simulink model "brayton_cycle_lstm_simplified_compare"  (R2023a)
settings: Solver=ode23t  StartTime=0.0  StopTime=100  RelTol=1e-3
PreLoadFcn:
  | combustor_volume = 0.001; % m^3
  | flow_area = 0.002; % m^2;
  | shaft_inertia = 0.1; % kg*m^2
  | mechanical_efficiency = 0.98; % 1
  | apu_shaft_speed = 6000; % rpm
  | 
  | % Compressor Map
  | 
  | compressor.beta_vector = [
  |      0, 0.1, 0.2, 0.3, 0.4, 0.5, 0.6, 0.7, 0.8, 0.9, 1.0];
  | 
  | compressor.corrected_speed_vector = [
  |     5000, 6000, 7000, 8000, 8500, 9000, 9500, 10000, 11000, 12000
  |     ]; % rpm
  | 
  | compressor.map.pressure_ratio = [
  |     0.1806    0.4817    0.8258    1.1561    1.4451    1.7002    2.0645    2.4086    2.6275    2.7527    2.8903
  |     0.2364    0.6303    1.0806    1.5128    1.8910    2.2247    2.7014    3.1517    3.4382    3.6019    3.7820
  |     0.2921    0.7790    1.3354    1.8695    2.3369    2.7493    3.3384    3.8948    4.2489    4.4512    4.6738
  |     0.4031    1.0748    1.8425    2.5795    3.2244    3.7934    4.6063    5.3740    5.8625    6.1417    6.4488
  |     0.5503    1.4673    2.5155    3.5216    4.4021    5.1789    6.2886    7.3368    8.0037    8.3849    8.8041
  |     0.7404    1.9745    3.3849    4.7388    5.9235    6.9688    8.4621    9.8725   10.7700   11.2829   11.8470
  |     0.9903    2.6407    4.5270    6.3378    7.9222    9.3203   11.3175   13.2037   14.4041   15.0900   15.8445
  |     1.2261    3.2697    5.6051    7.8472    9.8090   11.5400   14.0129   16.3483   17.8345   18.6838   19.6180
  |     1.2827    3.4206    5.8639    8.2094   10.2617   12.0726   14.6596   17.1029   18.6577   19.5462   20.5235
  |     1.3393    3.5715    6.1226    8.5716   10.7145   12.6053   15.3064   17.8575   19.4809   20.4086   21.4290]; % 1
  | 
  | compressor.map.corrected_mass_flow_rate = [
  |     0.0400    0.0400    0.0400    0.0399    0.0395    0.0389    0.0378    0.0363    0.0349    0.0340    0.0329
  |     0.0530    0.0530    0.0530    0.0527    0.0521    0.0513    0.0501    0.0481    0.0462    0.0449    0.0434
  |     0.0640    0.0640    0.0639    0.0635    0.0630    0.0623    0.0611    0.0589    0.0565    0.0549    0.0530
  |     0.1000    0.1000    0.0997    0.0991    0.0983    0.0974    0.0951    0.0906    0.0870    0.0846    0.0814
  |     0.1350    0.1350    0.1346    0.1340    0.1332    0.1324    0.1301    0.1258    0.1222    0.1197    0.1165
  |     0.1700    0.1699    0.1695    0.1688    0.1681    0.1673    0.1654    0.1620    0.1589    0.1562    0.1521
  |     0.2100    0.2097    0.2089    0.2077    0.2064    0.2051    0.2021    0.1978    0.1925    0.1882    0.1824
  |     0.2500    0.2498    0.2494    0.2488    0.2480    0.2472    0.2452    0.2414    0.2375    0.2338    0.2287
  |     0.2600    0.2599    0.2595    0.2589    0.2581    0.2574    0.2555    0.2516    0.2482    0.2453    0.2415
  |     0.2640    0.2639    0.2635    0.2629    0.2622    0.2616    0.2604    0.2580    0.2558    0.2542    0.2513]; % kg/s
  | 
  | compressor.map.efficiency = [
  |     0.3500    0.4200    0.4900    0.5600    0.5950    0.6300    0.6650    0.6860    0.6650    0.5600    0.4900
  |     0.3600    0.4320    0.5040    0.5760    0.6120    0.6480    0.6840    0.7056    0.6840    0.5760    0.5040
  |     0.3750    0.4500    0.5250    0.6000    0.6375    0.6750    0.7125    0.7350    0.7125    0.6000    0.5250
  |     0.3900    0.4680    0.5460    0.6240    0.6630    0.7020    0.7410    0.7644    0.7410    0.6240    0.5460
  |     0.4000    0.4800    0.5600    0.6400    0.6800    0.7200    0.7600    0.7840    0.7600    0.6400    0.5600
  |     0.4250    0.5100    0.5950    0.6800    0.7225    0.7650    0.8075    0.8330    0.8075    0.6800    0.5950
  |     0.4500    0.5400    0.6300    0.7200    0.7650    0.8100    0.8550    0.8820    0.8550    0.7200    0.6300
  |     0.4900    0.5880    0.6860    0.7840    0.8330    0.8820    0.9310    0.9604    0.9310    0.7840    0.6860
  |     0.4500    0.5400    0.6300    0.7200    0.7650    0.8100    0.8550    0.8820    0.8550    0.7200    0.6300
  |     0.4000    0.4800    0.5600    0.6400    0.6800    0.7200    0.7600    0.7840    0.7600    0.6400    0.5600]; % 1
  | 
  | compressor.reference_pressure = 0.101325; % MPa
  | compressor.reference_temperature = 288.15; % K
  | 
  | % Turbine Map
  | 
  | turbine.flow_map.pressure_ratio = [
  |     1.0010, 1.0050, 1.0101, 1.0204, 1.0309, 1.0417, 1.0526, 1.1111, 1.1765, 1.2500, 1.3333, 1.4286, 1.5385, 1.6667, 1.8182, 2.0000
  |     ]; %  1
  | turbine.flow_map.corrected_mass_flow_rate = [
  | ... (+17 lines)
model workspace (MAT data in the model file):
  rpm0 = 4800
  rpm_setpoint = [4000 4000 5000 5000 6000 6000 7000 7000 8000 8000 9000 9000 ... (19 elements, 1x19)]
  time_setpoint = [0 200 220 300 320 400 420 500 520 600 620 700 ... (19 elements, 1x19)]
undefined symbols (not defined in the file or in its folder): ix, scenario
libraries: fl_lib x32, nesl_utility x10, simulink x4, SimscapeFluids_lib x3, slpidlib x3, deeplib x3, SignalEditorBlockLib x1
(part 2 of 2)

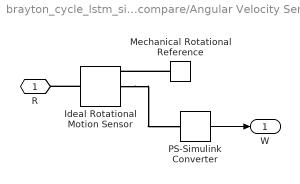
== system brayton_cycle_lstm_simplified_compare/Angular Velocity Sensor ==
  Ideal Rotational Motion Sensor : fl_lib/Mechanical/Mechanical Sensors/Ideal Rotational Motion Sensor  reference=foundation.enum.MeasurementReference.difference  acceleration_port=false  velocity_port=true  position_port=true  wrap_angle=simscape.enum.onoff.off  offset=0 rad
  Mechanical Rotational Reference : fl_lib/Mechanical/Rotational Elements/Mechanical Rotational Reference
  PS-Simulink Converter : nesl_utility/PS-Simulink Converter  PhysicalDomain=network_engine_domain  SubClassName=ps_output  LeftPortType=input  RightPortType=output  PseudoPeriodic=off  Frequencies=[]  VectorFormat=1-D array  Unit=rpm  AffineConversion=off
  R : PMIOPort  Side=Left
  W : Outport  VectorParamsAs1DForOutWhenUnconnected=off
  wires:
  PS-Simulink Converter/1 -> W/1
  connections:
  Ideal Rotational Motion Sensor/LConn1 -- R/RConn1
  Ideal Rotational Motion Sensor/RConn2 -- PS-Simulink Converter/LConn1
  Mechanical Rotational Reference/LConn1 -- Ideal Rotational Motion Sensor/RConn1

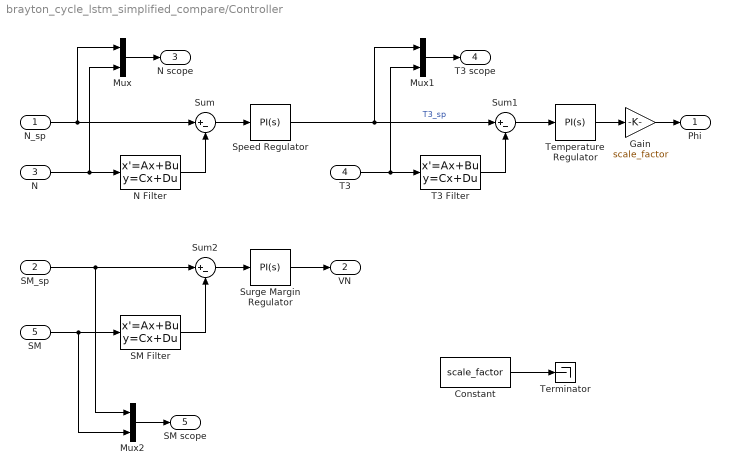
== system brayton_cycle_lstm_simplified_compare/Controller ==
  N_sp : Inport
  SM_sp : Inport  Port=2
  N : Inport  Port=3
  T3 : Inport  Port=4
  SM : Inport  Port=5
  Constant : Constant  Value=scale_factor
  Gain : Gain  Gain=scale_factor
  Mux : Mux  Inputs=2
  Mux1 : Mux  Inputs=2
  Mux2 : Mux  Inputs=2
  N Filter : StateSpace  A=-100  B=100  D=0  InitialCondition=10000
  SM Filter : StateSpace  A=-100  B=100  D=0  InitialCondition=0.25
  Speed Regulator : slpidlib/PID Controller  Controller=PI  Form=Ideal  TimeDomain=Continuous-time  UseExternalTs=off  SampleTime=-1  IntegratorMethod=Forward Euler  FilterMethod=Forward Euler  ControllerParametersSource=internal  P=0.5  I=1  UseKiTs=off  D=0  N=100  UseFilter=on  TunerSelectOption=Transfer Function Based (PID Tuner App)  InitialConditionSource=internal  InitialConditionForIntegrator=273.15  InitialConditionForFilter=0  DifferentiatorICPrevScaledInput=0  ExternalReset=none  TrackingMode=off  Kt=1  LimitOutput=on  SatLimitsSource=internal  UpperSaturationLimit=1800  LowerSaturationLimit=273.15  LinearizeAsGain=on  AntiWindupMode=back-calculation  Kb=1/0.5  LimitIntegrator=off  UpperIntegratorSaturationLimit=inf  LowerIntegratorSaturationLimit=-inf  POutMin=[]  POutMax=[]  IOutMin=[]  IOutMax=[]  DOutMin=[]  DOutMax=[]  NOutMin=[]  NOutMax=[]  SumOutMin=[]  SumOutMax=[]  SaturationOutMin=[]  SaturationOutMax=[]  PParamMin=[]  PParamMax=[]  IParamMin=[]  IParamMax=[]  DParamMin=[]  DParamMax=[]  NParamMin=[]  NParamMax=[]  KbParamMin=[]  KbParamMax=[]  KtParamMin=[]  KtParamMax=[]  KbOutMin=[]  KbOutMax=[]  KtOutMin=[]  KtOutMax=[]  IntegratorOutMin=[]  IntegratorOutMax=[]  FilterOutMin=[]  FilterOutMax=[]  SumI1OutMin=[]  SumI1OutMax=[]  SumI2OutMin=[]  SumI2OutMax=[]  SumI3OutMin=[]  SumI3OutMax=[]  SumI4OutMin=[]  SumI4OutMax=[]  SumDOutMin=[]  SumDOutMax=[]  DifferentiatorOutMin=[]  DifferentiatorOutMax=[]  FilterDiffOutCoefMin=[]  FilterDiffOutCoefMax=[]  ReciprocalOutMin=[]  ReciprocalOutMax=[]  SumDenOutMin=[]  SumDenOutMax=[]  SumNumOutMin=[]  SumNumOutMax=[]  DivideOutMin=[]  DivideOutMax=[]  UdiffTsProdOutMin=[]  UdiffTsProdOutMax=[]  NTsProdOutMin=[]  NTsProdOutMax=[]  UintegralTsProdOutMin=[]  UintegralTsProdOutMax=[]  UngainTsProdOutMin=[]  UngainTsProdOutMax=[]  ClampingZeroOutDataTypeStr=Inherit: Inherit via back propagation  ClampingZeroOutMin=[]  ClampingZeroOutMax=[]  FilterDenConstantOutDataTypeStr=Inherit: Inherit via back propagation  FilterDenConstantOutMin=[]  FilterDenConstantOutMax=[]  PCopyOutDataTypeStr=Inherit: Inherit via back propagation  PCopyOutMin=[]  PCopyOutMax=[]  NCopyOutDataTypeStr=Inherit: Inherit via back propagation  NCopyOutMin=[]  NCopyOutMax=[]  IntegratorContinuousStateAttributes=''  IntegratorStateMustResolveToSignalObject=off  IntegratorRTWStateStorageClass=Auto  FilterContinuousStateAttributes=''  FilterStateMustResolveToSignalObject=off  FilterRTWStateStorageClass=Auto  ParallelPVariant=Passthrough  IdealPVariant=InternalParameters  IVariant=InternalParameters  DVariant=Disabled  IntegratorVariant=Continuous  SatVariant=Enabled  AWVariant=BackCalculation  PCopyVariant=Disabled  TRVariant=Disabled  FdbkBlocksVariant=Forward  IdealPFdbkVariant=Disabled  SatFdbkVariant=Disabled  DerivativeFilterVariant=Disabled  NVariant=Disabled  NCopyVariant=Disabled_SignalSpec  FilterICVariant=Disabled  IntegratorICVariant=InternalICs  ExternalResetVariant=Disabled  TRSumVariant=Passthrough  SumFdbkVariant=Disabled  SumVariant=Sum_PI  TsampFilterVariant=InternalTs  TsampNgainVariant=Passthrough  TsampIntegralVariant=Disabled_SignalSpec  ExternalSaturationOutDataTypeStr=Inherit: Same as second input
  Sum : Sum  Inputs=|+-
  Sum1 : Sum  Inputs=|+-
  Sum2 : Sum  Inputs=|+-
  Surge Margin Regulator : slpidlib/PID Controller  Controller=PI  Form=Ideal  TimeDomain=Continuous-time  UseExternalTs=off  SampleTime=-1  IntegratorMethod=Forward Euler  FilterMethod=Forward Euler  ControllerParametersSource=internal  P=1  I=1  UseKiTs=off  D=0  N=100  UseFilter=on  TunerSelectOption=Transfer Function Based (PID Tuner App)  InitialConditionSource=internal  InitialConditionForIntegrator=0.15  InitialConditionForFilter=0  DifferentiatorICPrevScaledInput=0  ExternalReset=none  TrackingMode=off  Kt=1  LimitOutput=on  SatLimitsSource=internal  UpperSaturationLimit=1  LowerSaturationLimit=0.15  LinearizeAsGain=on  AntiWindupMode=back-calculation  Kb=1  LimitIntegrator=off  UpperIntegratorSaturationLimit=inf  LowerIntegratorSaturationLimit=-inf  POutMin=[]  POutMax=[]  IOutMin=[]  IOutMax=[]  DOutMin=[]  DOutMax=[]  NOutMin=[]  NOutMax=[]  SumOutMin=[]  SumOutMax=[]  SaturationOutMin=[]  SaturationOutMax=[]  PParamMin=[]  PParamMax=[]  IParamMin=[]  IParamMax=[]  DParamMin=[]  DParamMax=[]  NParamMin=[]  NParamMax=[]  KbParamMin=[]  KbParamMax=[]  KtParamMin=[]  KtParamMax=[]  KbOutMin=[]  KbOutMax=[]  KtOutMin=[]  KtOutMax=[]  IntegratorOutMin=[]  IntegratorOutMax=[]  FilterOutMin=[]  FilterOutMax=[]  SumI1OutMin=[]  SumI1OutMax=[]  SumI2OutMin=[]  SumI2OutMax=[]  SumI3OutMin=[]  SumI3OutMax=[]  SumI4OutMin=[]  SumI4OutMax=[]  SumDOutMin=[]  SumDOutMax=[]  DifferentiatorOutMin=[]  DifferentiatorOutMax=[]  FilterDiffOutCoefMin=[]  FilterDiffOutCoefMax=[]  ReciprocalOutMin=[]  ReciprocalOutMax=[]  SumDenOutMin=[]  SumDenOutMax=[]  SumNumOutMin=[]  SumNumOutMax=[]  DivideOutMin=[]  DivideOutMax=[]  UdiffTsProdOutMin=[]  UdiffTsProdOutMax=[]  NTsProdOutMin=[]  NTsProdOutMax=[]  UintegralTsProdOutMin=[]  UintegralTsProdOutMax=[]  UngainTsProdOutMin=[]  UngainTsProdOutMax=[]  ClampingZeroOutDataTypeStr=Inherit: Inherit via back propagation  ClampingZeroOutMin=[]  ClampingZeroOutMax=[]  FilterDenConstantOutDataTypeStr=Inherit: Inherit via back propagation  FilterDenConstantOutMin=[]  FilterDenConstantOutMax=[]  PCopyOutDataTypeStr=Inherit: Inherit via back propagation  PCopyOutMin=[]  PCopyOutMax=[]  NCopyOutDataTypeStr=Inherit: Inherit via back propagation  NCopyOutMin=[]  NCopyOutMax=[]  IntegratorContinuousStateAttributes=''  IntegratorStateMustResolveToSignalObject=off  IntegratorRTWStateStorageClass=Auto  FilterContinuousStateAttributes=''  FilterStateMustResolveToSignalObject=off  FilterRTWStateStorageClass=Auto  ParallelPVariant=Passthrough  IdealPVariant=InternalParameters  IVariant=InternalParameters  DVariant=Disabled  IntegratorVariant=Continuous  SatVariant=Enabled  AWVariant=BackCalculation  PCopyVariant=Disabled  TRVariant=Disabled  FdbkBlocksVariant=Forward  IdealPFdbkVariant=Disabled  SatFdbkVariant=Disabled  DerivativeFilterVariant=Disabled  NVariant=Disabled  NCopyVariant=Disabled_SignalSpec  FilterICVariant=Disabled  IntegratorICVariant=InternalICs  ExternalResetVariant=Disabled  TRSumVariant=Passthrough  SumFdbkVariant=Disabled  SumVariant=Sum_PI  TsampFilterVariant=InternalTs  TsampNgainVariant=Passthrough  TsampIntegralVariant=Disabled_SignalSpec  ExternalSaturationOutDataTypeStr=Inherit: Same as second input
  T3 Filter : StateSpace  A=-100  B=100  D=0  InitialCondition=288.15
  Temperature Regulator : slpidlib/PID Controller  Controller=PI  Form=Ideal  TimeDomain=Continuous-time  UseExternalTs=off  SampleTime=-1  IntegratorMethod=Forward Euler  FilterMethod=Forward Euler  ControllerParametersSource=internal  P=2  I=1  UseKiTs=off  D=0  N=100  UseFilter=on  TunerSelectOption=Transfer Function Based (PID Tuner App)  InitialConditionSource=internal  InitialConditionForIntegrator=0  InitialConditionForFilter=0  DifferentiatorICPrevScaledInput=0  ExternalReset=none  TrackingMode=off  Kt=1  LimitOutput=on  SatLimitsSource=internal  UpperSaturationLimit=500  LowerSaturationLimit=0  LinearizeAsGain=on  AntiWindupMode=back-calculation  Kb=1/2  LimitIntegrator=off  UpperIntegratorSaturationLimit=inf  LowerIntegratorSaturationLimit=-inf  POutMin=[]  POutMax=[]  IOutMin=[]  IOutMax=[]  DOutMin=[]  DOutMax=[]  NOutMin=[]  NOutMax=[]  SumOutMin=[]  SumOutMax=[]  SaturationOutMin=[]  SaturationOutMax=[]  PParamMin=[]  PParamMax=[]  IParamMin=[]  IParamMax=[]  DParamMin=[]  DParamMax=[]  NParamMin=[]  NParamMax=[]  KbParamMin=[]  KbParamMax=[]  KtParamMin=[]  KtParamMax=[]  KbOutMin=[]  KbOutMax=[]  KtOutMin=[]  KtOutMax=[]  IntegratorOutMin=[]  IntegratorOutMax=[]  FilterOutMin=[]  FilterOutMax=[]  SumI1OutMin=[]  SumI1OutMax=[]  SumI2OutMin=[]  SumI2OutMax=[]  SumI3OutMin=[]  SumI3OutMax=[]  SumI4OutMin=[]  SumI4OutMax=[]  SumDOutMin=[]  SumDOutMax=[]  DifferentiatorOutMin=[]  DifferentiatorOutMax=[]  FilterDiffOutCoefMin=[]  FilterDiffOutCoefMax=[]  ReciprocalOutMin=[]  ReciprocalOutMax=[]  SumDenOutMin=[]  SumDenOutMax=[]  SumNumOutMin=[]  SumNumOutMax=[]  DivideOutMin=[]  DivideOutMax=[]  UdiffTsProdOutMin=[]  UdiffTsProdOutMax=[]  NTsProdOutMin=[]  NTsProdOutMax=[]  UintegralTsProdOutMin=[]  UintegralTsProdOutMax=[]  UngainTsProdOutMin=[]  UngainTsProdOutMax=[]  ClampingZeroOutDataTypeStr=Inherit: Inherit via back propagation  ClampingZeroOutMin=[]  ClampingZeroOutMax=[]  FilterDenConstantOutDataTypeStr=Inherit: Inherit via back propagation  FilterDenConstantOutMin=[]  FilterDenConstantOutMax=[]  PCopyOutDataTypeStr=Inherit: Inherit via back propagation  PCopyOutMin=[]  PCopyOutMax=[]  NCopyOutDataTypeStr=Inherit: Inherit via back propagation  NCopyOutMin=[]  NCopyOutMax=[]  IntegratorContinuousStateAttributes=''  IntegratorStateMustResolveToSignalObject=off  IntegratorRTWStateStorageClass=Auto  FilterContinuousStateAttributes=''  FilterStateMustResolveToSignalObject=off  FilterRTWStateStorageClass=Auto  ParallelPVariant=Passthrough  IdealPVariant=InternalParameters  IVariant=InternalParameters  DVariant=Disabled  IntegratorVariant=Continuous  SatVariant=Enabled  AWVariant=BackCalculation  PCopyVariant=Disabled  TRVariant=Disabled  FdbkBlocksVariant=Forward  IdealPFdbkVariant=Disabled  SatFdbkVariant=Disabled  DerivativeFilterVariant=Disabled  NVariant=Disabled  NCopyVariant=Disabled_SignalSpec  FilterICVariant=Disabled  IntegratorICVariant=InternalICs  ExternalResetVariant=Disabled  TRSumVariant=Passthrough  SumFdbkVariant=Disabled  SumVariant=Sum_PI  TsampFilterVariant=InternalTs  TsampNgainVariant=Passthrough  TsampIntegralVariant=Disabled_SignalSpec  ExternalSaturationOutDataTypeStr=Inherit: Same as second input
  Terminator : Terminator
  Phi : Outport  VectorParamsAs1DForOutWhenUnconnected=off
  VN : Outport  Port=2  VectorParamsAs1DForOutWhenUnconnected=off
  N scope : Outport  Port=3  VectorParamsAs1DForOutWhenUnconnected=off
  T3 scope : Outport  Port=4  VectorParamsAs1DForOutWhenUnconnected=off
  SM scope : Outport  Port=5  VectorParamsAs1DForOutWhenUnconnected=off
  wires:
  N Filter/1 -> Sum/2
  Sum/1 -> Speed Regulator/1
  Sum1/1 -> Temperature Regulator/1
  T3 Filter/1 -> Sum1/2
  Sum2/1 -> Surge Margin Regulator/1
  SM Filter/1 -> Sum2/2
  N_sp/1 -> Sum/1, Mux/1
  N/1 -> N Filter/1, Mux/2
  Speed Regulator/1 -> Sum1/1, Mux1/1  "T3_sp"
  T3/1 -> T3 Filter/1, Mux1/2
  Temperature Regulator/1 -> Gain/1
  SM_sp/1 -> Sum2/1, Mux2/1
  SM/1 -> Mux2/2, SM Filter/1
  Surge Margin Regulator/1 -> VN/1
  Mux/1 -> N scope/1
  Mux1/1 -> T3 scope/1
  Mux2/1 -> SM scope/1
  Constant/1 -> Terminator/1
  Gain/1 -> Phi/1

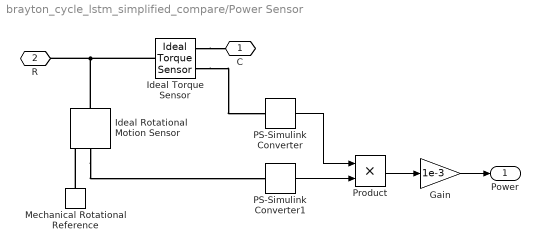
== system brayton_cycle_lstm_simplified_compare/Power Sensor ==
  Gain : Gain  Gain=1e-3
  Ideal Rotational Motion Sensor : fl_lib/Mechanical/Mechanical Sensors/Ideal Rotational Motion Sensor  reference=foundation.enum.MeasurementReference.difference  acceleration_port=false  velocity_port=true  position_port=true  wrap_angle=simscape.enum.onoff.off  offset=0 rad
  Ideal Torque Sensor : fl_lib/Mechanical/Mechanical Sensors/Ideal Torque Sensor
  Mechanical Rotational Reference : fl_lib/Mechanical/Rotational Elements/Mechanical Rotational Reference
  PS-Simulink Converter : nesl_utility/PS-Simulink Converter  PhysicalDomain=network_engine_domain  SubClassName=ps_output  LeftPortType=input  RightPortType=output  PseudoPeriodic=off  Frequencies=[]  VectorFormat=1-D array  Unit=N*m  AffineConversion=off
  PS-Simulink Converter1 : nesl_utility/PS-Simulink Converter  PhysicalDomain=network_engine_domain  SubClassName=ps_output  LeftPortType=input  RightPortType=output  PseudoPeriodic=off  Frequencies=[]  VectorFormat=1-D array  Unit=rad/s  AffineConversion=off
  Product : Product
  C : PMIOPort  Side=Left
  R : PMIOPort  Port=2  Side=Right
  Power : Outport  VectorParamsAs1DForOutWhenUnconnected=off
  wires:
  PS-Simulink Converter/1 -> Product/1
  PS-Simulink Converter1/1 -> Product/2
  Product/1 -> Gain/1
  Gain/1 -> Power/1
  connections:
  Ideal Torque Sensor/RConn1 -- C/RConn1
  Ideal Torque Sensor/RConn2 -- PS-Simulink Converter/LConn1
  Ideal Torque Sensor/LConn1 -- Ideal Rotational Motion Sensor/LConn1 -- R/RConn1
  Mechanical Rotational Reference/LConn1 -- Ideal Rotational Motion Sensor/RConn1
  Ideal Rotational Motion Sensor/RConn2 -- PS-Simulink Converter1/LConn1

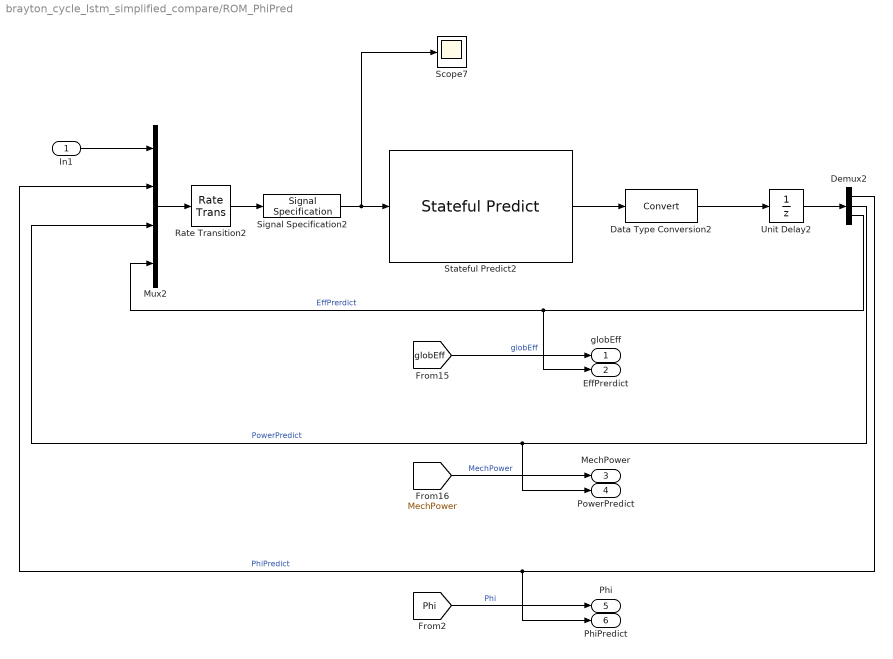
== system brayton_cycle_lstm_simplified_compare/ROM_PhiPred ==
  In1 : Inport
  Data Type Conversion2 : DataTypeConversion  SaturateOnIntegerOverflow=off  RndMeth=Floor
  Demux2 : Demux  Outputs=3
  Mux2 : Mux
  Rate Transition2 : RateTransition  OutPortSampleTime=0.1
  Scope7 : Scope
  Signal Specification2 : SignalSpecification  Dimensions=[4 1]
  Stateful Predict2 : deeplib/Stateful Predict  Network=Network from MAT-file  NetworkFunction=untitled  NetworkFilePath=C:\Users\imyrsini\OneDrive - MathWorks\Documents\Projects\AEprojects\LSTM Model Reduction\BraytonGasTurbSimplified_LSTMReduction\DL_backup\braytonLSTMNetThermo_SimplifiedPredictPhi.mat  InputDataFormats={'',''}  SampleTime=-1  ForceInterpretedSim=off  EnableDLNetwork=on
  Unit Delay2 : UnitDelay  InitialCondition=[0; 0; 0]  SampleTime=-1  HasFrameUpgradeWarning=on
  globEff : Outport
  EffPrerdict : Outport  Port=2
  MechPower : Outport  Port=3
  PowerPredict : Outport  Port=4
  Phi : Outport  Port=5
  PhiPredict : Outport  Port=6
  wires:
  Mux2/1 -> Rate Transition2/1
  Signal Specification2/1 -> Scope7/1, Stateful Predict2/1
  In1/1 -> Mux2/1
  Demux2/1 -> PhiPredict/1, Mux2/2  "PhiPredict"
  Unit Delay2/1 -> Demux2/1
  Demux2/3 -> EffPrerdict/1, Mux2/4  "EffPrerdict"
  Data Type Conversion2/1 -> Unit Delay2/1
  Rate Transition2/1 -> Signal Specification2/1
  Stateful Predict2/1 -> Data Type Conversion2/1
  [Phi] -> Phi/1  "Phi"
  Demux2/2 -> PowerPredict/1, Mux2/3  "PowerPredict"
  [globEff] -> globEff/1  "globEff"
  [MechPower] -> MechPower/1  "MechPower"

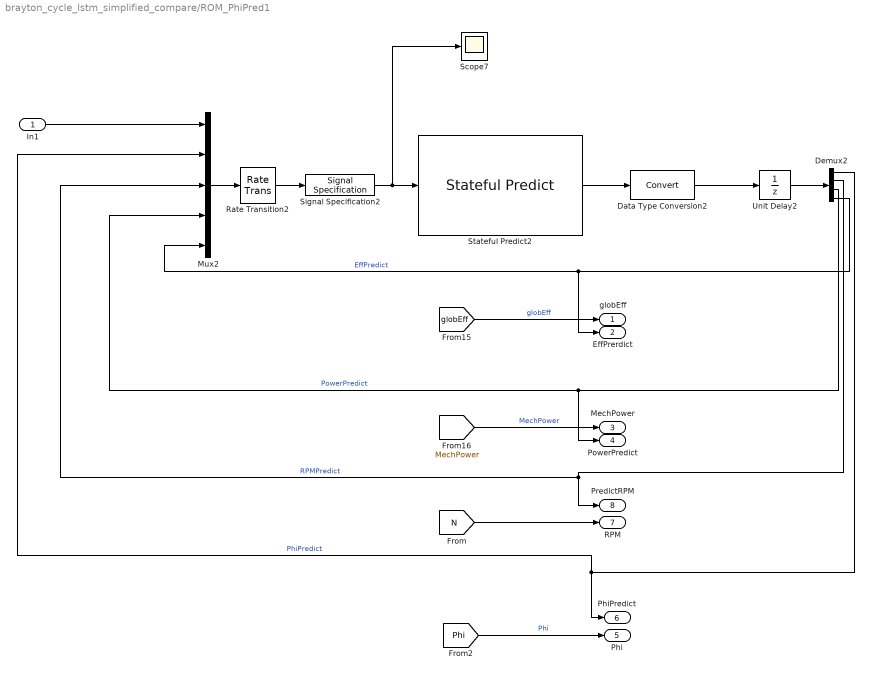
== system brayton_cycle_lstm_simplified_compare/ROM_PhiPred1 ==
  In1 : Inport
  Data Type Conversion2 : DataTypeConversion  SaturateOnIntegerOverflow=off  RndMeth=Floor
  Demux2 : Demux
  Mux2 : Mux  Inputs=5
  Rate Transition2 : RateTransition  OutPortSampleTime=0.1
  Scope7 : Scope
  Signal Specification2 : SignalSpecification  Dimensions=[5 1]
  Stateful Predict2 : deeplib/Stateful Predict  Network=Network from MAT-file  NetworkFunction=untitled  NetworkFilePath=C:\Users\imyrsini\OneDrive - MathWorks\Documents\Projects\AEprojects\LSTM Model Reduction\BraytonGasTurbSimplified_LSTMReduction\DL_backup\braytonLSTMNetThermo_LR003_stairsFixed_Mixed.mat  InputDataFormats={'',''}  SampleTime=-1  ForceInterpretedSim=off  EnableDLNetwork=on
  Unit Delay2 : UnitDelay  InitialCondition=[0; rpm0; 0; 0]  SampleTime=-1  HasFrameUpgradeWarning=on
  globEff : Outport
  EffPrerdict : Outport  Port=2
  MechPower : Outport  Port=3
  PowerPredict : Outport  Port=4
  Phi : Outport  Port=5
  PhiPredict : Outport  Port=6
  RPM : Outport  Port=7
  PredictRPM : Outport  Port=8
  wires:
  [MechPower] -> MechPower/1  "MechPower"
  [globEff] -> globEff/1  "globEff"
  [Phi] -> Phi/1  "Phi"
  Stateful Predict2/1 -> Data Type Conversion2/1
  Rate Transition2/1 -> Signal Specification2/1
  Data Type Conversion2/1 -> Unit Delay2/1
  Unit Delay2/1 -> Demux2/1
  In1/1 -> Mux2/1
  Signal Specification2/1 -> Stateful Predict2/1, Scope7/1
  Mux2/1 -> Rate Transition2/1
  Demux2/1 -> PhiPredict/1, Mux2/2  "PhiPredict"
  Demux2/2 -> Mux2/3, PredictRPM/1  "RPMPredict"
  [N] -> RPM/1
  Demux2/3 -> Mux2/4, PowerPredict/1  "PowerPredict"
  Demux2/4 -> Mux2/5, EffPrerdict/1  "EffPredict"

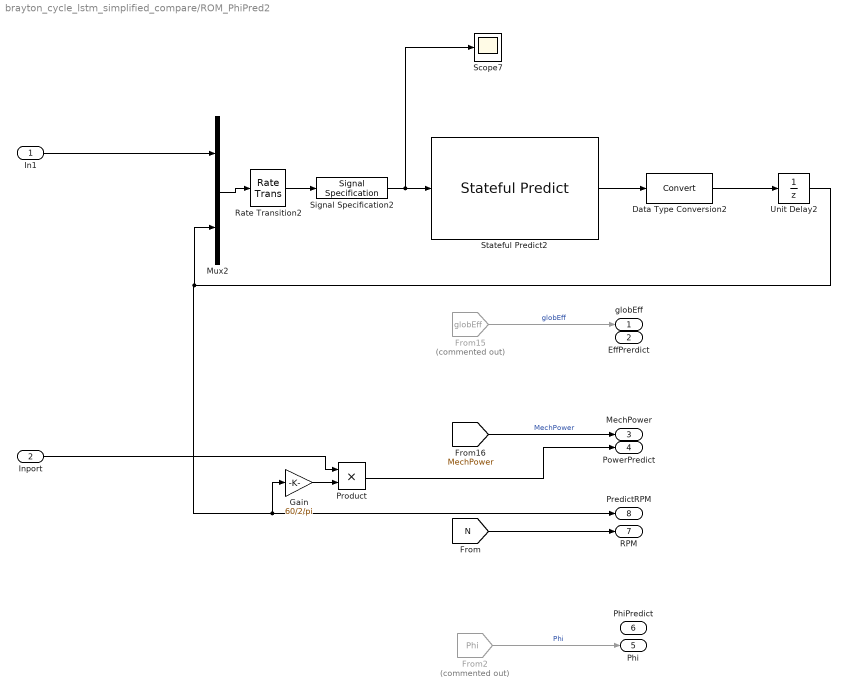
== system brayton_cycle_lstm_simplified_compare/ROM_PhiPred2 ==
  In1 : Inport
  Inport : Inport  Port=2
  Data Type Conversion2 : DataTypeConversion  SaturateOnIntegerOverflow=off  RndMeth=Floor
  From15 : From  Commented=on  GotoTag=globEff  TagVisibility=global
  From2 : From  Commented=on  GotoTag=Phi  TagVisibility=global
  Gain : Gain  Gain=60/2/pi
  Mux2 : Mux  Inputs=2
  Product : Product
  Rate Transition2 : RateTransition  OutPortSampleTime=0.1
  Scope7 : Scope
  Signal Specification2 : SignalSpecification  Dimensions=[2 1]
  Stateful Predict2 : deeplib/Stateful Predict  Network=Network from MAT-file  NetworkFunction=untitled  NetworkFilePath=C:\Users\imyrsini\OneDrive - MathWorks\Documents\Projects\AEprojects\LSTM Model Reduction\BraytonGasTurbSimplified_LSTMReduction\DL_backup\braytonLSTMNetThermo_ShartTrainLimitiedConstant.mat  InputDataFormats={'',''}  SampleTime=-1  ForceInterpretedSim=off  EnableDLNetwork=on
  Unit Delay2 : UnitDelay  InitialCondition=[ 0]  SampleTime=-1  HasFrameUpgradeWarning=on
  globEff : Outport
  EffPrerdict : Outport  Port=2
  MechPower : Outport  Port=3
  PowerPredict : Outport  Port=4
  Phi : Outport  Port=5
  PhiPredict : Outport  Port=6
  RPM : Outport  Port=7
  PredictRPM : Outport  Port=8
  wires:
  Mux2/1 -> Rate Transition2/1
  Signal Specification2/1 -> Scope7/1, Stateful Predict2/1
  In1/1 -> Mux2/1
  Data Type Conversion2/1 -> Unit Delay2/1
  Rate Transition2/1 -> Signal Specification2/1
  Stateful Predict2/1 -> Data Type Conversion2/1
  From2/1 -> Phi/1  "Phi"
  From15/1 -> globEff/1  "globEff"
  [MechPower] -> MechPower/1  "MechPower"
  Inport/1 -> Product/1
  Gain/1 -> Product/2
  Product/1 -> PowerPredict/1
  [N] -> RPM/1
  Unit Delay2/1 -> Gain/1, PredictRPM/1, Mux2/2

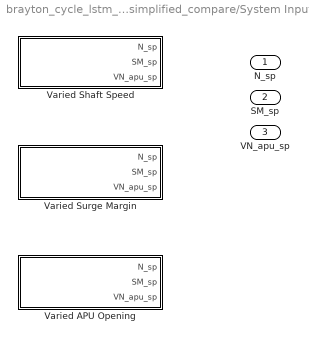
== system brayton_cycle_lstm_simplified_compare/System Inputs ==
  Varied APU Opening : Subsystem  VariantControl=Varied APU Opening
  Varied Shaft Speed : Subsystem  VariantControl=Varied Shaft Speed
  Varied Surge Margin : Subsystem  VariantControl=Varied Surge Margin
  N_sp : Outport
  SM_sp : Outport  Port=2
  VN_apu_sp : Outport  Port=3

== system brayton_cycle_lstm_simplified_compare/T,s 1 ==
  Absolute Reference (G) : fl_lib/Gas/Elements/Absolute Reference (G)
      settings: InternalSimscapePortConfiguration="{\"Bottom\":[],\"Left\":[{\"id\":\"A\",\"label\":\"\",\"type\":\"foundation.gas.gas\"}],\"Right\":[],\"Top\":[]}"
  Pressure & Temperature Sensor (G) : fl_lib/Gas/Sensors/Pressure & Temperature Sensor (G)  reference=foundation.enum.MeasurementReference.difference  pressure=true  pressure_spec=foundation.enum.PressureMeasementSpec.Absolute  temperature=true
      settings: InternalSimscapePortConfiguration="{\"Bottom\":[{\"id\":\"T\",\"label\":\"T\",\"type\":\"output\"}],\"Left\":[{\"id\":\"A\",\"label\":\"A\",\"type\":\"foundation.gas.gas\"}],\"Right\":[{\"id\":\"B\",\"label\":\"B\",\"type\":\"foundation.gas.gas\"},{\"id\":\"P\",\"label\":\"P\",\"type\":\"output\"}],\"Top\":[]}"
  Thermodynamic Properties Sensor (G) : fl_lib/Gas/Sensors/Thermodynamic Properties Sensor (G)  enthalpy=true  density=true  specific_heat=true  entropy=true  s_std=3.8635 kJ/kg/K  p_std=0.101325 MPa  T_std=293.15 K
      settings: InternalSimscapePortConfiguration="{\"Bottom\":[{\"id\":\"CP\",\"label\":\"cp\",\"type\":\"output\"},{\"id\":\"S\",\"label\":\"s\",\"type\":\"output\"}],\"Left\":[{\"id\":\"A\",\"label\":\"A\",\"type\":\"foundation.gas.gas\"}],\"Right\":[{\"id\":\"H\",\"label\":\"h\",\"type\":\"output\"},{\"id\":\"RHO\",\"label\":\"ρ\",\"type\":\"output\"}],\"Top\":[]}"
  A : PMIOPort  Side=Left
  connections:
  Absolute Reference (G)/LConn1 -- Pressure & Temperature Sensor (G)/RConn1
  Thermodynamic Properties Sensor (G)/LConn1 -- A/RConn1 -- Pressure & Temperature Sensor (G)/LConn1

== system brayton_cycle_lstm_simplified_compare/T,s 2 ==
  Absolute Reference (G) : fl_lib/Gas/Elements/Absolute Reference (G)
      settings: InternalSimscapePortConfiguration="{\"Bottom\":[],\"Left\":[{\"id\":\"A\",\"label\":\"\",\"type\":\"foundation.gas.gas\"}],\"Right\":[],\"Top\":[]}"
  Pressure & Temperature Sensor (G) : fl_lib/Gas/Sensors/Pressure & Temperature Sensor (G)  reference=foundation.enum.MeasurementReference.difference  pressure=true  pressure_spec=foundation.enum.PressureMeasementSpec.Absolute  temperature=true
      settings: InternalSimscapePortConfiguration="{\"Bottom\":[{\"id\":\"T\",\"label\":\"T\",\"type\":\"output\"}],\"Left\":[{\"id\":\"A\",\"label\":\"A\",\"type\":\"foundation.gas.gas\"}],\"Right\":[{\"id\":\"B\",\"label\":\"B\",\"type\":\"foundation.gas.gas\"},{\"id\":\"P\",\"label\":\"P\",\"type\":\"output\"}],\"Top\":[]}"
  Thermodynamic Properties Sensor (G) : fl_lib/Gas/Sensors/Thermodynamic Properties Sensor (G)  enthalpy=true  density=true  specific_heat=true  entropy=true  s_std=3.8635 kJ/kg/K  p_std=0.101325 MPa  T_std=293.15 K
      settings: InternalSimscapePortConfiguration="{\"Bottom\":[{\"id\":\"CP\",\"label\":\"cp\",\"type\":\"output\"},{\"id\":\"S\",\"label\":\"s\",\"type\":\"output\"}],\"Left\":[{\"id\":\"A\",\"label\":\"A\",\"type\":\"foundation.gas.gas\"}],\"Right\":[{\"id\":\"H\",\"label\":\"h\",\"type\":\"output\"},{\"id\":\"RHO\",\"label\":\"ρ\",\"type\":\"output\"}],\"Top\":[]}"
  A : PMIOPort  Side=Left
  connections:
  Pressure & Temperature Sensor (G)/LConn1 -- A/RConn1 -- Thermodynamic Properties Sensor (G)/LConn1
  Absolute Reference (G)/LConn1 -- Pressure & Temperature Sensor (G)/RConn1

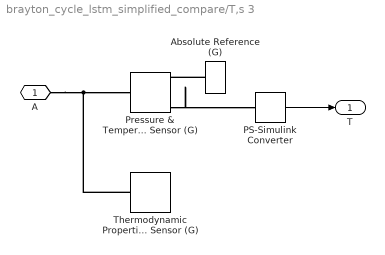
== system brayton_cycle_lstm_simplified_compare/T,s 3 ==
  Absolute Reference (G) : fl_lib/Gas/Elements/Absolute Reference (G)
      settings: InternalSimscapePortConfiguration="{\"Bottom\":[],\"Left\":[{\"id\":\"A\",\"label\":\"\",\"type\":\"foundation.gas.gas\"}],\"Right\":[],\"Top\":[]}"
  PS-Simulink Converter : nesl_utility/PS-Simulink Converter  PhysicalDomain=network_engine_domain  SubClassName=ps_output  LeftPortType=input  RightPortType=output  PseudoPeriodic=off  Frequencies=[]  VectorFormat=1-D array  Unit=K  AffineConversion=on
  Pressure & Temperature Sensor (G) : fl_lib/Gas/Sensors/Pressure & Temperature Sensor (G)  reference=foundation.enum.MeasurementReference.difference  pressure=true  pressure_spec=foundation.enum.PressureMeasementSpec.Absolute  temperature=true
      settings: InternalSimscapePortConfiguration="{\"Bottom\":[{\"id\":\"T\",\"label\":\"T\",\"type\":\"output\"}],\"Left\":[{\"id\":\"A\",\"label\":\"A\",\"type\":\"foundation.gas.gas\"}],\"Right\":[{\"id\":\"B\",\"label\":\"B\",\"type\":\"foundation.gas.gas\"},{\"id\":\"P\",\"label\":\"P\",\"type\":\"output\"}],\"Top\":[]}"
  Thermodynamic Properties Sensor (G) : fl_lib/Gas/Sensors/Thermodynamic Properties Sensor (G)  enthalpy=true  density=true  specific_heat=true  entropy=true  s_std=3.8635 kJ/kg/K  p_std=0.101325 MPa  T_std=293.15 K
      settings: InternalSimscapePortConfiguration="{\"Bottom\":[{\"id\":\"CP\",\"label\":\"cp\",\"type\":\"output\"},{\"id\":\"S\",\"label\":\"s\",\"type\":\"output\"}],\"Left\":[{\"id\":\"A\",\"label\":\"A\",\"type\":\"foundation.gas.gas\"}],\"Right\":[{\"id\":\"H\",\"label\":\"h\",\"type\":\"output\"},{\"id\":\"RHO\",\"label\":\"ρ\",\"type\":\"output\"}],\"Top\":[]}"
  A : PMIOPort  Side=Left
  T : Outport  VectorParamsAs1DForOutWhenUnconnected=off
  wires:
  PS-Simulink Converter/1 -> T/1
  connections:
  A/RConn1 -- Thermodynamic Properties Sensor (G)/LConn1 -- Pressure & Temperature Sensor (G)/LConn1
  Absolute Reference (G)/LConn1 -- Pressure & Temperature Sensor (G)/RConn1
  Pressure & Temperature Sensor (G)/RConn3 -- PS-Simulink Converter/LConn1

== system brayton_cycle_lstm_simplified_compare/T,s 4 ==
  Absolute Reference (G) : fl_lib/Gas/Elements/Absolute Reference (G)
      settings: InternalSimscapePortConfiguration="{\"Bottom\":[],\"Left\":[{\"id\":\"A\",\"label\":\"\",\"type\":\"foundation.gas.gas\"}],\"Right\":[],\"Top\":[]}"
  Pressure & Temperature Sensor (G) : fl_lib/Gas/Sensors/Pressure & Temperature Sensor (G)  reference=foundation.enum.MeasurementReference.difference  pressure=true  pressure_spec=foundation.enum.PressureMeasementSpec.Absolute  temperature=true
      settings: InternalSimscapePortConfiguration="{\"Bottom\":[{\"id\":\"T\",\"label\":\"T\",\"type\":\"output\"}],\"Left\":[{\"id\":\"A\",\"label\":\"A\",\"type\":\"foundation.gas.gas\"}],\"Right\":[{\"id\":\"B\",\"label\":\"B\",\"type\":\"foundation.gas.gas\"},{\"id\":\"P\",\"label\":\"P\",\"type\":\"output\"}],\"Top\":[]}"
  Thermodynamic Properties Sensor (G) : fl_lib/Gas/Sensors/Thermodynamic Properties Sensor (G)  enthalpy=true  density=true  specific_heat=true  entropy=true  s_std=3.8635 kJ/kg/K  p_std=0.101325 MPa  T_std=293.15 K
      settings: InternalSimscapePortConfiguration="{\"Bottom\":[{\"id\":\"CP\",\"label\":\"cp\",\"type\":\"output\"},{\"id\":\"S\",\"label\":\"s\",\"type\":\"output\"}],\"Left\":[{\"id\":\"A\",\"label\":\"A\",\"type\":\"foundation.gas.gas\"}],\"Right\":[{\"id\":\"H\",\"label\":\"h\",\"type\":\"output\"},{\"id\":\"RHO\",\"label\":\"ρ\",\"type\":\"output\"}],\"Top\":[]}"
  A : PMIOPort  Side=Left
  connections:
  Absolute Reference (G)/LConn1 -- Pressure & Temperature Sensor (G)/RConn1
  Thermodynamic Properties Sensor (G)/LConn1 -- A/RConn1 -- Pressure & Temperature Sensor (G)/LConn1

== system brayton_cycle_lstm_simplified_compare/T,s 5 ==
  Absolute Reference (G) : fl_lib/Gas/Elements/Absolute Reference (G)
      settings: InternalSimscapePortConfiguration="{\"Bottom\":[],\"Left\":[{\"id\":\"A\",\"label\":\"\",\"type\":\"foundation.gas.gas\"}],\"Right\":[],\"Top\":[]}"
  Pressure & Temperature Sensor (G) : fl_lib/Gas/Sensors/Pressure & Temperature Sensor (G)  reference=foundation.enum.MeasurementReference.difference  pressure=true  pressure_spec=foundation.enum.PressureMeasementSpec.Absolute  temperature=true
      settings: InternalSimscapePortConfiguration="{\"Bottom\":[{\"id\":\"T\",\"label\":\"T\",\"type\":\"output\"}],\"Left\":[{\"id\":\"A\",\"label\":\"A\",\"type\":\"foundation.gas.gas\"}],\"Right\":[{\"id\":\"B\",\"label\":\"B\",\"type\":\"foundation.gas.gas\"},{\"id\":\"P\",\"label\":\"P\",\"type\":\"output\"}],\"Top\":[]}"
  Thermodynamic Properties Sensor (G) : fl_lib/Gas/Sensors/Thermodynamic Properties Sensor (G)  enthalpy=true  density=true  specific_heat=true  entropy=true  s_std=3.8635 kJ/kg/K  p_std=0.101325 MPa  T_std=293.15 K
      settings: InternalSimscapePortConfiguration="{\"Bottom\":[{\"id\":\"CP\",\"label\":\"cp\",\"type\":\"output\"},{\"id\":\"S\",\"label\":\"s\",\"type\":\"output\"}],\"Left\":[{\"id\":\"A\",\"label\":\"A\",\"type\":\"foundation.gas.gas\"}],\"Right\":[{\"id\":\"H\",\"label\":\"h\",\"type\":\"output\"},{\"id\":\"RHO\",\"label\":\"ρ\",\"type\":\"output\"}],\"Top\":[]}"
  A : PMIOPort  Side=Left
  connections:
  Pressure & Temperature Sensor (G)/LConn1 -- A/RConn1 -- Thermodynamic Properties Sensor (G)/LConn1
  Absolute Reference (G)/LConn1 -- Pressure & Temperature Sensor (G)/RConn1

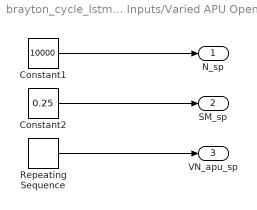
== system brayton_cycle_lstm_simplified_compare/System Inputs/Varied APU Opening ==
  Constant1 : Constant  Value=10000
  Constant2 : Constant  Value=0.25
  Repeating Sequence : simulink/Sources/Repeating Sequence  rep_seq_t=[0 200 210 300 310 400 410 500 510 600 610 700 710 800 810 900 910 1000 1100]  rep_seq_y=[0.25 0.25 0.3 0.3 0.35 0.35 0.4 0.4 0.45 0.45 0.5 0.5 0.55 0.55 0.6 0.6 0.65 0.65 0.65]
  N_sp : Outport
  SM_sp : Outport  Port=2
  VN_apu_sp : Outport  Port=3
  wires:
  Constant1/1 -> N_sp/1
  Constant2/1 -> SM_sp/1
  Repeating Sequence/1 -> VN_apu_sp/1

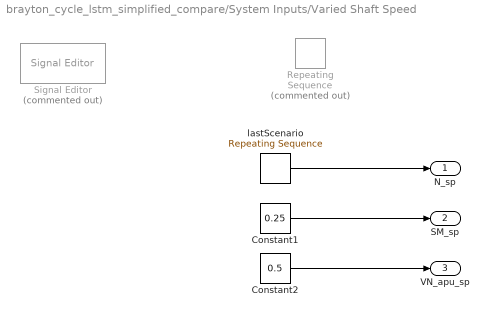
== system brayton_cycle_lstm_simplified_compare/System Inputs/Varied Shaft Speed ==
  Constant1 : Constant  Value=0.25
  Constant2 : Constant  Value=0.5
  Repeating Sequence : simulink/Sources/Repeating Sequence  Commented=on  rep_seq_t=time_setpoint  rep_seq_y=rpm_setpoint
  Signal Editor : SignalEditorBlockLib/Signal Editor  Commented=on  FileName=stairShaftSpeed_11100_4100_st_1000.mat  ActiveScenario=shaftSpeedRef  ActiveSignal=stairShaftSpeed_11100_4100  IsBus=off  OutputBusObjectStr=Bus: BusObject  SampleTime=0  Interpolate=off  ZeroCross=off  OutputAfterFinalValue=Setting to zero  Unit=inherit  PreserveSignalName=on  ApplySigPropsToAllScenarios=on
  lastScenario : simulink/Sources/Repeating Sequence  rep_seq_t=scenario{ix}.shaftSpeedRef{1}.Values.Time'  rep_seq_y=scenario{ix}.shaftSpeedRef{1}.Values.Data'
  N_sp : Outport
  SM_sp : Outport  Port=2
  VN_apu_sp : Outport  Port=3
  wires:
  Constant1/1 -> SM_sp/1
  Constant2/1 -> VN_apu_sp/1
  lastScenario/1 -> N_sp/1

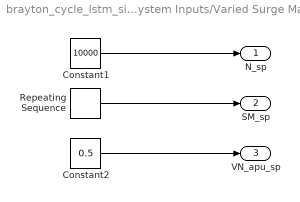
== system brayton_cycle_lstm_simplified_compare/System Inputs/Varied Surge Margin ==
  Constant1 : Constant  Value=10000
  Constant2 : Constant  Value=0.5
  Repeating Sequence : simulink/Sources/Repeating Sequence  rep_seq_t=[0 200 210 300 310 400 410 500 510 600 610 700 710 800 810 900 910 1000 1100]  rep_seq_y=[0.9 0.9 0.8 0.8 0.7 0.7 0.6 0.6 0.5 0.5 0.4 0.4 0.3 0.3 0.2 0.2 0.1 0.1 0.1]
  N_sp : Outport
  SM_sp : Outport  Port=2
  VN_apu_sp : Outport  Port=3
  wires:
  Constant2/1 -> VN_apu_sp/1
  Constant1/1 -> N_sp/1
  Repeating Sequence/1 -> SM_sp/1
